simulink model "pitch_corrector"  (R2019a)
settings: Solver=FixedStepAuto  StartTime=0.0  StopTime=inf  RelTol=1e-3  EnableMultiTasking=on
libraries: embdlinuxlib x2, dspindex x1
settings Model: SimulationMode=external  Creator=Antonio  LastModifiedBy=cresp
settings SolverCC: PositivePriorityOrder=on
settings DataIOCC: ReturnWorkspaceOutputs=off
settings OptimizationCC: EnhancedBackFolding=on  PassReuseOutputArgsAs=Individual arguments  MaxStackSize=64  OptimizeBlockOrder=speed  DifferentSizesBufferReuse=on  OptimizationCustomize=off
settings DebuggingCC: ParameterTunabilityLossMsg=error  PregeneratedLibrarySubsystemCodeDiagnostic=none  ArithmeticOperatorsInVariantConditions=warning
settings HardwareCC: ProdBitPerPointer=32  ProdBitPerSizeT=32  ProdBitPerPtrDiffT=32  ProdLargestAtomicInteger=Long  ProdLargestAtomicFloat=Double  ProdWordSize=32  ProdHWDeviceType=ARM Compatible->ARM Cortex
settings SFSimCC: SimUseLocalCustomCode=off  MATLABDynamicMemAlloc=off
settings RTWCC: SystemTargetFile=ert.tlc  HardwareBoard=Raspberry Pi  TLCOptions="-aInlineSetEventsForThisBaseRateFcn=TLC_FALSE -aSuppressMultiTaskScheduler=TLC_FALSE  -aRateBasedStepFcn=0"  TemplateMakefile=ert_default_tmf  GenerateReport=on  RTWUseLocalCustomCode=off  Toolchain=GNU GCC Raspberry Pi  BuildConfiguration=Faster Runs  IncludeHyperlinkInReport=on  LaunchReport=on  GenerateTraceInfo=on  GenerateTraceReport=on  GenerateTraceReportSl=on  GenerateTraceReportSf=on  GenerateTraceReportEml=on
settings CodeAppCC: ForceParamTrailComments=on  IgnoreCustomStorageClasses=off  OperatorAnnotations=on  SimulinkDataObjDesc=on  SFDataObjDesc=on  InsertBlockDesc=on
settings ERTTargetCC: SupportVariableSizeSignals=on

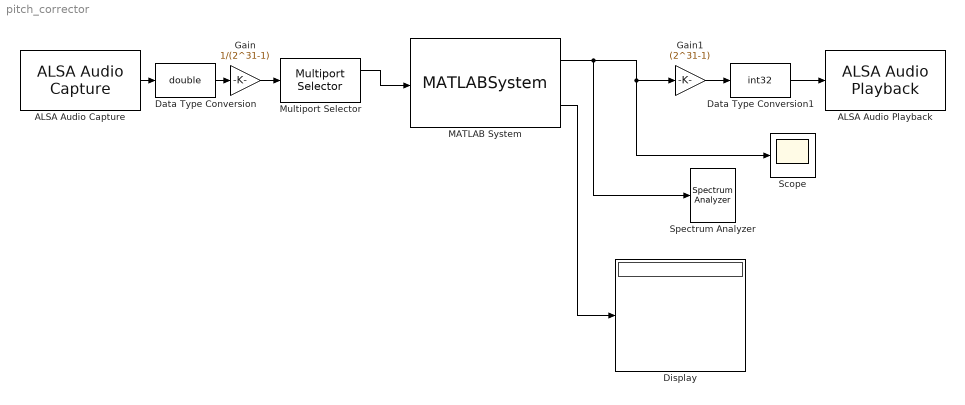
== system pitch_corrector ==
  ALSA Audio Capture : embdlinuxlib/ALSA Audio Capture  deviceStr='default'  DataBitDepth=32-bit integer  numberOfChannels=2  sampleRateEnum=16000  frameSize=512  QueueDuration=0  blockPlatform=Raspberry Pi
      settings: SourceProductName=Simulink Coder Support Package for BeagleBone Blue Hardware  SourceProductBaseCode=SC_BEAGLEBONE_BLUE
  ALSA Audio Playback : embdlinuxlib/ALSA Audio Playback  deviceStr='default'  sampleRateEnum=16000  queueDuration=0  blockPlatform=Raspberry Pi
      settings: SourceProductName=Simulink Coder Support Package for BeagleBone Blue Hardware  SourceProductBaseCode=SC_BEAGLEBONE_BLUE
  Data Type Conversion : DataTypeConversion  OutDataTypeStr=double
  Data Type Conversion1 : DataTypeConversion  OutDataTypeStr=int32
  Display : Display
  Gain : Gain  Gain=1/(2^31-1)
  Gain1 : Gain  Gain=(2^31-1)
  MATLAB System : MATLABSystem  System=main  Fs=16000  SimulateUsing=Code generation
      mask Type: main
      mask Display:
      | disp('main');
      | port_label('input',1,'in');
      | port_label('output',1,'out');
      | port_label('output',2,'debug');
  Multiport Selector : dspindex/Multiport Selector  rowsOrCols=Columns  idxCellArray={ 1,2 }  idxErrMode=Clip Index
  Scope : Scope
  Spectrum Analyzer : SpectrumAnalyzer
  wires:
  Multiport Selector/1 -> MATLAB System/1
  Gain/1 -> Multiport Selector/1
  ALSA Audio Capture/1 -> Data Type Conversion/1
  Data Type Conversion/1 -> Gain/1
  MATLAB System/1 -> Spectrum Analyzer/1, Gain1/1, Scope/1
  Data Type Conversion1/1 -> ALSA Audio Playback/1
  Gain1/1 -> Data Type Conversion1/1
  MATLAB System/2 -> Display/1
